simulink model "SistemaMassaMollaSmorzatore"  (R2020b)
settings: Solver=VariableStepAuto  StartTime=0.0  StopTime=10.0  RelTol=1e-3
undefined symbols (not defined in the file or in its folder): D, K, M, sigbuilder_block
libraries: simulink x1
settings Model: Creator=loryb  LastModifiedBy=loryb

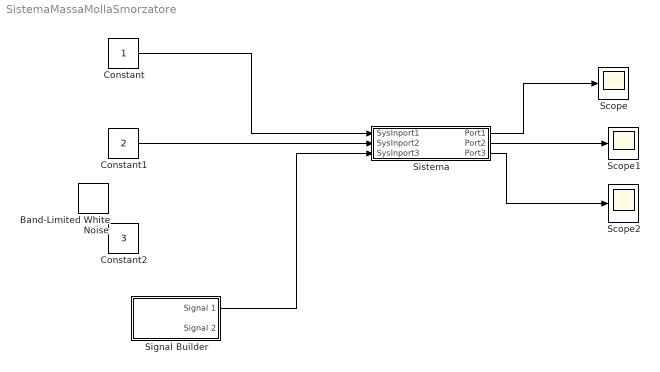
== system SistemaMassaMollaSmorzatore ==
  Band-Limited White Noise : simulink/Sources/Band-Limited White Noise  Cov=[0.1]  Ts=0.1  seed=[23341]
  Constant : Constant
  Constant1 : Constant  Value=2
  Constant2 : Constant  Value=3
  Scope : Scope
  Scope1 : Scope
  Scope2 : Scope
  Signal Builder : Subsystem  Tag=STV Subsys  LoadFcn=sigbuilder_block('load');  StartFcn=sigbuilder_block('start');  StopFcn=sigbuilder_block('stop');  ClipboardFcn=sigbuilder_block('clipboard');  mask(Sigbuilder block){tuvar=[0:10]}
      mask help: Simulink:masks:SigbuilderBlock_MD
      mask init:
      | if ~strcmp(get_param(bdroot(gcbh),'SimulationStatus'),'stopped') tuvar = sigbuilder_block('maskInit'); end
      settings: CopyFcn=sigbuilder_block('copy');  DeleteFcn=sigbuilder_block('delete');  ModelCloseFcn=sigbuilder_block('modelClose');  PreSaveFcn=sigbuilder_block('preSave');  PauseFcn=sigbuilder_block('pause');  ContinueFcn=sigbuilder_block('continue');  NameChangeFcn=sigbuilder_block('namechange');  OpenFcn=sigbuilder_block('open',[106.5 108.75 550.5 399.75 ]);  CloseFcn=sigbuilder_block('close');
      mask Display: plot(0, 0, 100, 100,[2, 2, 32, 32, 2], [68, 8, 8, 68, 68],[32, 2], [38, 38], [32, 19, 2],[53, 60, 44], [32, 17, 17, 2],[16, 16, 31, 31]);txt = getActiveGroup(gcbh);text(2, 100, txt,'verticalAlignment', 'top');
  "Sistema " : Subsystem  mask(Differential Equation Editor (DEE)){}
      settings: OpenFcn=diffeqed
      mask Display: disp('Differential Equation\n Editor')
  wires:
  Constant/1 -> "Sistema "/1(SysInport1)
  Constant1/1 -> "Sistema "/2(SysInport2)
  "Sistema "/1(Port1) -> Scope/1
  "Sistema "/2(Port2) -> Scope1/1
  "Sistema "/3(Port3) -> Scope2/1
  Signal Builder/1(Signal 1) -> "Sistema "/3(SysInport3)

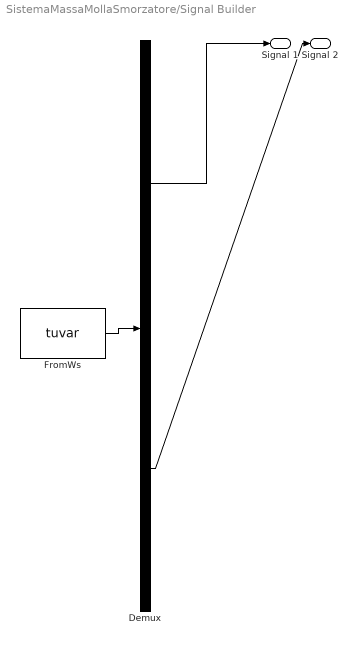
== system SistemaMassaMollaSmorzatore/Signal Builder ==
  Demux : Demux  Tag=STV Demux  Outputs=2
      settings: DisplayOption=none
  FromWs : FromWorkspace  Tag=STV FromWs  VariableName=tuvar
      SigBuilderData=|
      | common.afterFinalStr = 'Extrapolate'
      | common.sampleTime = 0
      | dataSet.timeRange = [0 10]
      | dataSet.name = 'Group 1'
      | sbobj.Groups.Name = 'Group 1'
      | sbobj.Groups.Signals(1).Name = 'Signal 1'
      | sbobj.Groups.Signals(1).XData = [0 4 4 6 6 10]
      | sbobj.Groups.Signals(1).YData = [0.41 0.41 1 1 0 0]
      | sbobj.Groups.Signals(2).Name = 'Signal 2'
      | sbobj.Groups.Signals(2).XData = [0 10]
      | sbobj.Groups.Signals(2).YData = [0 0]
  Signal 1 : Outport  Tag=STV Outport
  Signal 2 : Outport  Tag=STV Outport  Port=2
  wires:
  Demux/1 -> Signal 1/1
  FromWs/1 -> Demux/1
  Demux/2 -> Signal 2/1

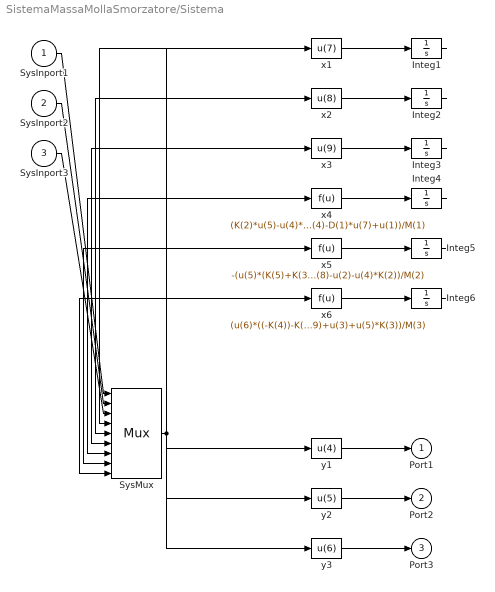
== system SistemaMassaMollaSmorzatore/Sistema  ==
  SysInport1 : Inport
  SysInport2 : Inport  Port=2
  SysInport3 : Inport  Port=3
  Integ{1..6} (6 alike) : Integrator
  SysMux : Mux  Inputs=9
  x1 : Fcn  Expr=u(7)
  x2 : Fcn  Expr=u(8)
  x3 : Fcn  Expr=u(9)
  x4 : Fcn  Expr=(K(2)*u(5)-u(4)*K(2)-K(1)*u(4)-D(1)*u(7)+u(1))/M(1)
  x5 : Fcn  Expr=-(u(5)*(K(5)+K(3)+K(2))-K(3)*u(6)+D(2)*u(8)-u(2)-u(4)*K(2))/M(2)
  x6 : Fcn  Expr=(u(6)*((-K(4))-K(3))-D(3)*u(9)+u(3)+u(5)*K(3))/M(3)
  y1 : Fcn  Expr=u(4)
  y2 : Fcn  Expr=u(5)
  y3 : Fcn  Expr=u(6)
  Port1 : Outport
  Port2 : Outport  Port=2
  Port3 : Outport  Port=3
  wires:
  SysInport1/1 -> SysMux/1
  SysInport2/1 -> SysMux/2
  SysInport3/1 -> SysMux/3
  SysMux/1 -> x1/1, x2/1, x3/1, x4/1, x5/1, x6/1, y1/1, y2/1, y3/1
  x1/1 -> Integ1/1
  Integ1/1 -> SysMux/4
  x2/1 -> Integ2/1
  Integ2/1 -> SysMux/5
  x3/1 -> Integ3/1
  Integ3/1 -> SysMux/6
  x4/1 -> Integ4/1
  Integ4/1 -> SysMux/7
  x5/1 -> Integ5/1
  Integ5/1 -> SysMux/8
  x6/1 -> Integ6/1
  Integ6/1 -> SysMux/9
  y1/1 -> Port1/1
  y2/1 -> Port2/1
  y3/1 -> Port3/1
